simulink model "openloop_gaslift"  (R2023a)
settings: Solver=ode15s  StartTime=0.0  StopTime=par.simulation_time  FixedStep=par.sample_time  RelTol=1e-3
values from neighbouring files (symbols this model uses):
  par = function_parameters_openloop_gaslift    [main_openloop_gaslift.m]
settings Model: Creator=aslik  LastModifiedBy=aslik
settings DataIOCC: SaveOutput=off  InspectSignalLogs=on  SaveTime=off  ReturnWorkspaceOutputs=off  DatasetSignalFormat=timetable

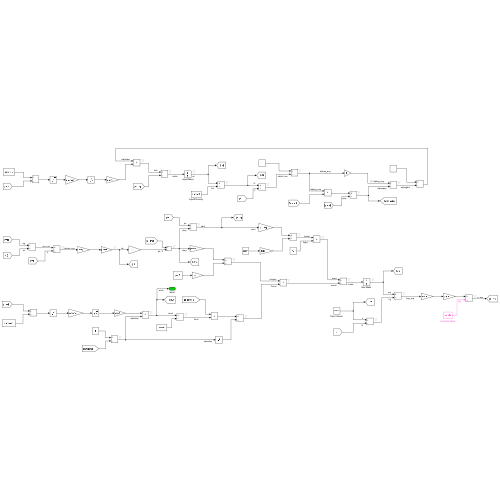
[thumbnail: Simulink's stored preview of the top-level diagram]
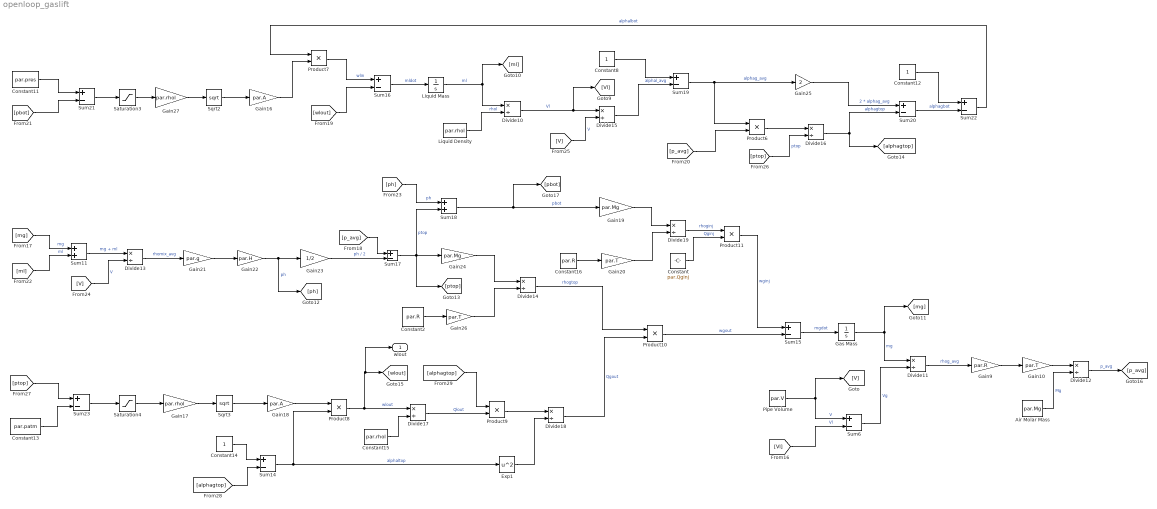
== system openloop_gaslift ==
  Air Molar Mass : Constant  Value=par.Mg  OutDataTypeStr=double
  Constant : Constant  Value=par.Qginj
  Constant11 : Constant  Value=par.pres  OutDataTypeStr=double
  Constant12 : Constant  OutDataTypeStr=double
  Constant13 : Constant  Value=par.patm  OutDataTypeStr=double
  Constant14 : Constant  OutDataTypeStr=double
  Constant15 : Constant  Value=par.rhol  OutDataTypeStr=double
  Constant16 : Constant  Value=par.R  OutDataTypeStr=double
  Constant2 : Constant  Value=par.R  OutDataTypeStr=double
  Constant8 : Constant  OutDataTypeStr=double
  Divide{10..19} (10 alike) : Product  Inputs=*/
  Exp1 : Math  Operator=square
  Gain10 : Gain  Gain=par.T
  Gain16 : Gain  Gain=par.A
  Gain17 : Gain  Gain=par.rhol
  Gain18 : Gain  Gain=par.A
  Gain19 : Gain  Gain=par.Mg
  Gain20 : Gain  Gain=par.T
  Gain21 : Gain  Gain=par.g
  Gain22 : Gain  Gain=par.H
  Gain23 : Gain  Gain=1/2
  Gain24 : Gain  Gain=par.Mg
  Gain25 : Gain  Gain=2
  Gain26 : Gain  Gain=par.T
  Gain27 : Gain  Gain=par.rhol
  Gain9 : Gain  Gain=par.R
  "Gas Mass " : Integrator  InitialCondition=par.mg0  LowerSaturationLimit=0  ContinuousStateAttributes='mg'
  Liquid Density : Constant  Value=par.rhol  OutDataTypeStr=double
  Liquid Mass : Integrator  InitialCondition=par.ml0  LowerSaturationLimit=0  ContinuousStateAttributes='ml'
  Pipe Volume : Constant  Value=par.V  OutDataTypeStr=double
  Product{6..11} (6 alike) : Product
  Saturation3 : Saturate  UpperLimit=inf  LowerLimit=0
  Saturation4 : Saturate  UpperLimit=inf  LowerLimit=0
  Sqrt2 : Sqrt
  Sqrt3 : Sqrt
  Sum11 : Sum
  Sum{6,14..17,19..23} (10 alike) : Sum  Inputs=+-
  Sum18 : Sum
  wlout : Outport
  wires:
  Air Molar Mass/1 -> Divide12/2  "Mg"
  Divide11/1 -> Gain9/1  "rhog_avg"
  Sum15/1 -> "Gas Mass "/1  "mgdot"
  Gain21/1 -> Gain22/1
  Divide13/1 -> Gain21/1  "rhomix_avg"
  "Gas Mass "/1 -> [mg], Divide11/1  "mg"
  Sum22/1 -> Product7/1  "alphalbot"
  Pipe Volume/1 -> [V], Sum6/1  "V"
  Product8/1 -> wlout/1, [wlout], Divide17/1  "wlout"
  Gain19/1 -> Divide19/1
  Sqrt2/1 -> Gain16/1
  [wlout] -> Sum16/2
  Divide10/1 -> Divide15/1, [Vl]  "Vl"
  Sum17/1 -> Gain24/1, Sum18/2, [ptop]  "ptop"
  Constant15/1 -> Divide17/2
  Constant13/1 -> Sum23/2
  Sum21/1 -> Saturation3/1
  Gain18/1 -> Product8/1
  Sqrt3/1 -> Gain18/1
  Sum14/1 -> Product8/2, Exp1/1  "alphaltop"
  Constant/1 -> Product11/2  "Qginj"
  Product10/1 -> Sum15/2  "wgout"
  Exp1/1 -> Divide18/2
  Constant12/1 -> Sum22/1
  Liquid Mass/1 -> [ml], Divide10/1  "ml"
  [ptop] -> Divide16/2  "ptop"
  Sum6/1 -> Divide11/2  "Vg"
  Saturation4/1 -> Gain17/1
  Sum23/1 -> Saturation4/1
  Gain10/1 -> Divide12/1
  Product7/1 -> Sum16/1  "wlin"
  Gain22/1 -> [ph], Gain23/1  "ph"
  Sum11/1 -> Divide13/1  "mg + ml"
  Constant2/1 -> Gain26/1
  Gain26/1 -> Divide14/2
  [alphagtop] -> Product9/1
  [mg] -> Sum11/1  "mg"
  [p_avg] -> Product6/2
  Sum19/1 -> Product6/1, Gain25/1  "alphag_avg"
  [ph] -> Sum18/1  "ph"
  Sum16/1 -> Liquid Mass/1  "mldot"
  Divide15/1 -> Sum19/2  "alphal_avg"
  Divide18/1 -> Product10/2  "Qgout"
  Gain27/1 -> Sqrt2/1
  Constant14/1 -> Sum14/1
  Divide12/1 -> [p_avg]  "p_avg"
  Gain24/1 -> Divide14/1
  Product11/1 -> Sum15/1  "wginj"
  Gain25/1 -> Sum20/1  "2 * alphag_avg"
  Constant8/1 -> Sum19/1
  Saturation3/1 -> Gain27/1
  Product9/1 -> Divide18/1
  Gain9/1 -> Gain10/1
  Sum20/1 -> Sum22/2  "alphagbot"
  [ml] -> Sum11/2  "ml"
  [pbot] -> Sum21/2
  Product6/1 -> Divide16/1
  Divide17/1 -> Product9/2  "Qlout"
  [ptop] -> Sum23/1
  Divide16/1 -> [alphagtop], Sum20/2  "alphagtop"
  [V] -> Divide13/2  "V"
  Constant11/1 -> Sum21/1
  Liquid Density/1 -> Divide10/2  "rhol"
  [alphagtop] -> Sum14/2
  Gain16/1 -> Product7/2
  [p_avg] -> Sum17/1
  [Vl] -> Sum6/2  "Vl"
  Sum18/1 -> [pbot], Gain19/1  "pbot"
  Divide14/1 -> Product10/1  "rhogtop"
  Gain17/1 -> Sqrt3/1
  Gain20/1 -> Divide19/2
  Divide19/1 -> Product11/1  "rhoginj"
  [V] -> Divide15/2  "V"
  Constant16/1 -> Gain20/1
  Gain23/1 -> Sum17/2  "ph / 2"
